simulink model "Junctions7"  (Simulink 5.0)
settings: Solver=ode45  StartTime=0.0  StopTime=10.0  RelTol=1e-3
settings Model: Creator=scaife  LastModifiedBy=scaife  ExtModeAutoUpdateStatusClock=off

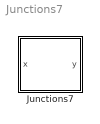
== system Junctions7 ==
  Junctions7 : Stateflow chart

== stateflow chart Junctions7 ==
  state A
  state B
  A -> (junction 5) : [x==0]{y--}
  A -> (junction 5) : [x<>0]{y++}
  (junction 5) -> B : [x<2]
  (default) -> A
  data: x input int32; y output int32
